simulink model "Control_de_corriente"  (R2021a)
settings: Solver=VariableStepAuto  StartTime=0.0  StopTime=10.0  RelTol=1e-3
undefined symbols (not defined in the file): lambda_m, Ld, Lq, Pp, R0, Rd, Rq, Rs
settings Model: Creator=fhlla  LastModifiedBy=fhlla

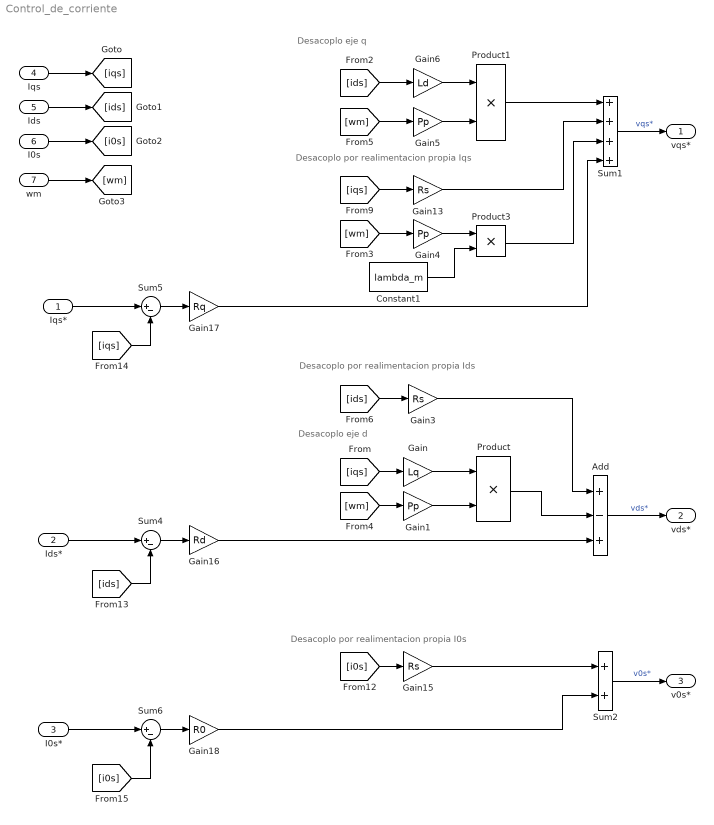
== system Control_de_corriente ==
  note: Desacoplo eje d
  note: Desacoplo por realimentacion propia I0s
  note: Desacoplo por realimentacion propia Iqs
  note: Desacoplo eje q
  note: Desacoplo por realimentacion propia Ids
  Iqs* : Inport
  Ids* : Inport  Port=2
  I0s* : Inport  Port=3
  Iqs : Inport  Port=4
  Ids : Inport  Port=5
  I0s : Inport  Port=6
  wm : Inport  Port=7
  Add : Sum  Inputs=+-+
  Constant1 : Constant  Value=lambda_m
  Gain : Gain  Gain=Lq
  Gain1 : Gain  Gain=Pp
  Gain13 : Gain  Gain=Rs
  Gain15 : Gain  Gain=Rs
  Gain16 : Gain  Gain=Rd
  Gain17 : Gain  Gain=Rq
  Gain18 : Gain  Gain=R0
  Gain3 : Gain  Gain=Rs
  Gain4 : Gain  Gain=Pp
  Gain5 : Gain  Gain=Pp
  Gain6 : Gain  Gain=Ld
  Product : Product
  Product1 : Product
  Product3 : Product
  Sum1 : Sum  Inputs=++++
  Sum2 : Sum
  Sum4 : Sum  Inputs=|+-
  Sum5 : Sum  Inputs=|+-
  Sum6 : Sum  Inputs=|+-
  vqs* : Outport
  vds* : Outport  Port=2
  v0s* : Outport  Port=3
  wires:
  Product1/1 -> Sum1/1
  wm/1 -> [wm]
  Sum1/1 -> vqs*/1  "vqs*"
  Product/1 -> Add/2
  [iqs] -> Gain/1
  Add/1 -> vds*/1  "vds*"
  Sum4/1 -> Gain16/1
  Constant1/1 -> Product3/2
  Gain4/1 -> Product3/1
  [i0s] -> Gain15/1
  [iqs] -> Sum5/2
  [wm] -> Gain5/1
  I0s/1 -> [i0s]
  Gain5/1 -> Product1/2
  Gain15/1 -> Sum2/1
  Sum5/1 -> Gain17/1
  Gain18/1 -> Sum2/2
  Gain17/1 -> Sum1/4
  [ids] -> Gain3/1
  Sum2/1 -> v0s*/1  "v0s*"
  [iqs] -> Gain13/1
  Ids*/1 -> Sum4/1
  Iqs*/1 -> Sum5/1
  Gain13/1 -> Sum1/2
  [i0s] -> Sum6/2
  Gain16/1 -> Add/3
  Product3/1 -> Sum1/3
  Gain/1 -> Product/1
  Gain1/1 -> Product/2
  Sum6/1 -> Gain18/1
  [wm] -> Gain1/1
  [wm] -> Gain4/1
  [ids] -> Gain6/1
  [ids] -> Sum4/2
  Iqs/1 -> [iqs]
  Ids/1 -> [ids]
  Gain6/1 -> Product1/1
  Gain3/1 -> Add/1
  I0s*/1 -> Sum6/1
